simulink model "model"  (R2018b)
settings: Solver=VariableStepAuto  StartTime=0.0  StopTime=Tsim  RelTol=1e-3
values from neighbouring files (symbols this model uses):
  alfa_b_1 = -1    [init.m]
  alfa_b_3 = 0.0066    [init.m]
  b2_ref = 1.541e-5    (= 1.541e-05)    [init.m]
  b3_ref = 2.805e-2    (= 0.02805)    [init.m]
  b_0 = 1.07    [init.m]
  b_1_ref = 3.503e-3    (= 0.003503)    [init.m]
  beta_b1 = 2.157    [init.m]
  beta_c2 = 4.54    [init.m]
  c_0_ref = 75.64    [init.m]
  c_2_ref = 3.9193e-3    (= 0.0039193)    [init.m]
  d_0_ref = 75.1    [init.m]
  d_3 = 0.46    [init.m]
  E_a_b2 = -42800    [init.m]
  E_a_b3 = 42800    [init.m]
  E_a_b_1 = 35392    [init.m]
  E_a_c0 = 2224    [init.m]
  E_a_c2 = -48260    [init.m]
  E_a_d_0_1 = 4126    [init.m]
  E_a_d_0_2 = 9.752e6    (= 9752000)    [init.m]
  F = 96485    [init.m]
  gamma_b_1 = 2.472    [init.m]
  R_ug = 8.314    [init.m]
  T_ref = 298.15    [init.m]
  tau_b_3 = 5    [init.m]
  theta = 0.135    [init.m]
  U_neg_ref = 0.08    [init.m]
  V_ref = 3.7    [init.m]
undefined symbols (not defined in the file or in its folder): magnitude
settings Model: Creator=Pedro  LastModifiedBy=Pedro

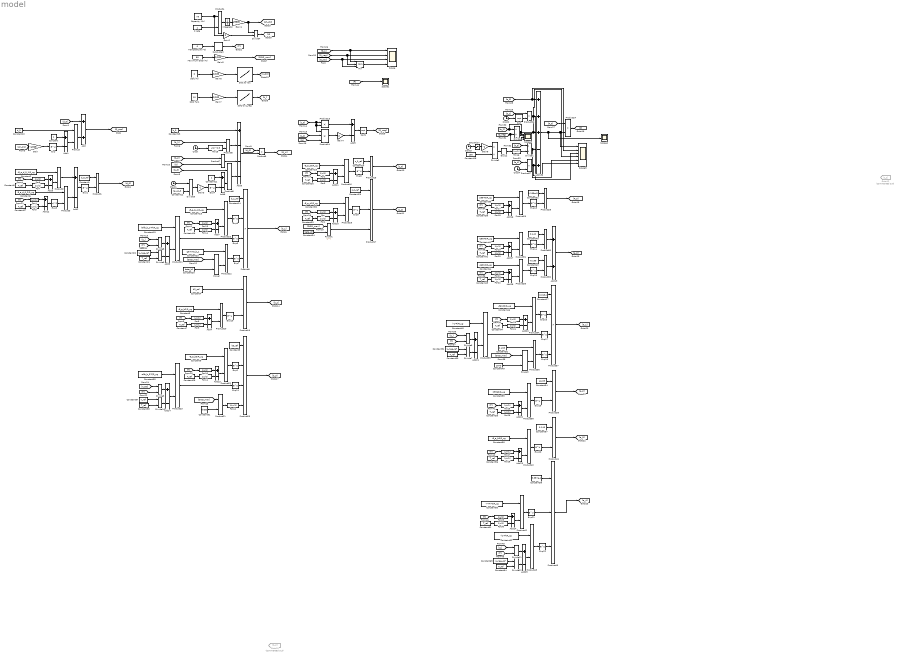
== system model ==
  Add : Sum
  Add{1..4,6..14,16..18,20..25} (22 alike) : Sum  Inputs=+-
  Add15 : Sum  Inputs=+++-+
  Add19 : Sum
  Add5 : Sum  Inputs=+---
  C rate : Constant
  Capacity (Ah) : Constant  Value=75
  Clock{,1..4} (5 alike) : Clock
  Constant : Constant
  Constant1 : Constant  Value=d_0_ref
  Constant10 : Constant  Value=d_3
  Constant11 : Constant
  Constant12 : Constant  Value=tau_b_3
  Constant13 : Constant  Value=b_0
  Constant14 : Constant  Value=b_1_ref
  Constant15 : Constant  Value=-E_a_b_1/R_ug
  Constant{3,7,16,21,26..28,33,38..39,42,45,47,50,53,56,61,64} (18 alike) : Constant  Value=T_ref
  Constant17 : Constant  Value=0.0134
  Constant18 : Constant  Value=100
  Constant19 : Constant  Value=(alfa_b_1*F)/R_ug
  Constant2 : Constant  Value=-E_a_d_0_1/R_ug
  Constant20 : Constant  Value=beta_b1
  Constant22 : Constant  Value=U_neg_ref
  Constant23 : Constant  Value=gamma_b_1
  Constant24 : Constant  Value=c_0_ref
  Constant25 : Constant  Value=-E_a_c0/R_ug  VectorParams1D=off
  Constant29 : Constant  Value=c_2_ref
  Constant30 : Constant  Value=-E_a_c2/R_ug  VectorParams1D=off
  Constant31 : Constant  Value=theta
  Constant32 : Constant  Value=1.155e-3
  Constant34 : Constant  Value=beta_c2
  Constant35 : Constant  Value=alfa_b_3*F/R_ug
  Constant36 : Constant  Value=28640/R_ug  VectorParams1D=off
  Constant37 : Constant  Value=V_ref
  Constant4 : Constant  Value=b2_ref
  Constant40 : Constant  Value=0.442
  Constant41 : Constant  Value=-28640/R_ug  VectorParams1D=off
  Constant43 : Constant  Value=-0.199
  Constant44 : Constant  Value=46010/R_ug  VectorParams1D=off
  Constant46 : Constant  Value=-36100/R_ug
  Constant48 : Constant  Value=(-1*F)/R_ug
  Constant49 : Constant  Value=1870
  Constant5 : Constant  Value=-E_a_b2/R_ug  VectorParams1D=off
  Constant51 : Constant  Value=U_neg_ref
  Constant52 : Constant  Value=2.433
  Constant54 : Constant  Value=46.05
  Constant55 : Constant  Value=29360/R_ug
  Constant57 : Constant  Value=0.145
  Constant58 : Constant  Value=-E_a_b3/R_ug
  Constant59 : Constant  Value=5.357e-4
  Constant6 : Constant  Value=E_a_d_0_2/R_ug
  Constant60 : Constant  Value=-77470/R_ug
  Constant62 : Constant  Value=(-1*F)/R_ug
  Constant65 : Constant  Value=U_neg_ref
  Constant8 : Constant  Value=b3_ref
  Constant9 : Constant  Value=-E_a_b3/R_ug
  Divide{,1..12} (13 alike) : Product  Inputs=*/
  Exp{,1..2,4..22} (22 alike) : Math  SaturateOnIntegerOverflow=on
  Exp3 : Math  Operator=magnitude^2  SaturateOnIntegerOverflow=on
  Fcn{,1..11,13..14,17..30} (28 alike) : Fcn  Expr=1/u(1)
  Fcn12 : Fcn  Expr=1+u(1)
  Fcn15 : Fcn  Expr=u(1)^0.5
  Fcn16 : Fcn  Expr=1-u(1)
  Gain : Gain  Gain=-1/228
  Gain1 : Gain  Gain=1/3600
  Gain2 : Gain  Gain=2
  Gain3 : Gain  Gain=-1
  Gain4 : Gain  Gain=2
  Gain5 : Gain  Gain=1/100
  Gain6 : Gain  Gain=1/100
  Gain7 : Gain  Gain=1/100
  Gain8 : Gain  Gain=-1
  Goto12 : Goto  Commented=on  GotoTag=c_2
  Goto15 : Goto  Commented=on  GotoTag=b_2
  Integrator : Integrator
  Maximum DOD (%) : Constant  Value=80
  Min : MinMax  Inputs=3
  Power : Math  Operator=pow  SaturateOnIntegerOverflow=on
  Power1 : Math  Operator=pow  SaturateOnIntegerOverflow=on
  Power2 : Math  Operator=pow  SaturateOnIntegerOverflow=on
  Product{,1..8,10..13,15..16,18..24,26..36,38..43} (39 alike) : Product
  Product14 : Product  Inputs=3
  Product17 : Product  Inputs=3
  Product25 : Product  Inputs=4
  Product37 : Product  Inputs=4
  Product45 : Product  Inputs=3
  Product9 : Product  Inputs=4
  SOC (%) : Constant  Value=0
  SOC (%)1 : Constant  Value=10
  SOC to U_neg : Lookup_n-D  NumberOfTableDimensions=1  BreakpointsForDimension1=[0 0.1 0.2 0.3 0.4 0.5 0.6 0.7 0.8 0.9 1.0]  Table=[1.2868 0.2420 0.1818 0.1488 0.1297 0.1230 0.1181 0.1061 0.0925 0.0876 0.0859]  InternalRulePriority=Speed  RndMeth=Simplest  InputSameDT=on
  SOC to Voc : Lookup_n-D  NumberOfTableDimensions=1  BreakpointsForDimension1=[0 0.1 0.2 0.3 0.4 0.5 0.6 0.7 0.8 0.9 1.0]  Table=[3.0000 3.4679 3.5394 3.5950 3.6453 3.6876 3.7469 3.8400 3.9521 4.0668 4.1934]  InternalRulePriority=Speed  RndMeth=Simplest  InputSameDT=on
  Saturation : Saturate  UpperLimit=inf  LowerLimit=1
  Scope : Scope  NumInputPorts=4
  Scope1 : Scope
  Scope2 : Scope
  Scope3 : Scope  NumInputPorts=3
  Scope5 : Scope  NumInputPorts=6
  Sqrt : Sqrt  SaturateOnIntegerOverflow=on
  Sqrt1 : Sqrt  SaturateOnIntegerOverflow=on
  Subsystem : Subsystem
  Temperature (°C) : Constant  Value=0
  wires:
  Constant10/1 -> Product/1
  Add1/1 -> Product/2
  Constant/1 -> Add1/1
  Exp/1 -> Add1/2
  Gain/1 -> Exp/1
  [Ah_dis] -> Gain/1
  Product/1 -> Add/2
  Add/1 -> [Q_pos]  "Positive electrode  site-limited capacity"
  Constant1/1 -> Product1/1
  Exp1/1 -> Product1/2
  Add2/1 -> Exp1/1
  Product1/1 -> [d_0]  "Increase in  capacity at BOL"
  Product2/1 -> Add2/1
  Product3/1 -> Add2/2
  Constant2/1 -> Product2/1
  Add12/1 -> Exp3/1
  Exp3/1 -> Product3/2
  [Q_pos] -> Min/3, Scope/3  "Q_pos"
  Integrator/1 -> Gain1/1
  Subsystem/1(°K) -> [T]
  Gain1/1 -> Divide4/1, [Ah_dis]
  C rate/1 -> Product4/2
  [d_0] -> Add/1
  Temperature (°C)/1 -> Subsystem/1(°C)
  Constant6/1 -> Product3/1
  Product4/1 -> Integrator/1
  Capacity (Ah)/1 -> Gain2/1, Product4/1
  Product5/1 -> [Q_Li]  "Li-limited  capacity"
  [d_0] -> Product5/1
  Add5/1 -> Product5/2
  Constant13/1 -> Add5/1
  Product6/1 -> Add5/2
  [b_1] -> Product6/1
  Fcn15/1 -> Product6/2
  Gain2/1 -> Divide4/2
  Product7/1 -> Add5/3
  [b_2] -> Product7/1
  [N] -> Product7/2
  [b_3] -> Product8/1
  Gain3/1 -> Exp4/1
  Constant11/1 -> Add6/1
  Add6/1 -> Product8/2
  Product8/1 -> Add5/4
  Exp4/1 -> Add6/2
  Divide5/1 -> Gain3/1
  Constant12/1 -> Divide5/2
  Product9/1 -> [b_1]  "SEI growth with calendar time"
  Constant14/1 -> Product9/1
  Exp5/1 -> Product9/2
  Constant15/1 -> Product10/1
  Product10/1 -> Exp5/1
  Product11/1 -> Exp6/1
  Constant21/1 -> Divide9/2
  [T] -> Divide8/2
  Constant22/1 -> Divide9/1
  Add8/1 -> Product11/2
  Constant19/1 -> Product11/1
  Divide9/1 -> Add8/2
  [U_] -> Divide8/1
  Divide8/1 -> Add8/1
  Constant23/1 -> Product12/1
  Power/1 -> Product12/2
  [DOD_max] -> Power/1
  Constant20/1 -> Power/2
  Sqrt1/1 -> [Q_neg]
  Add9/1 -> Sqrt1/1
  [c_0] -> Product14/1, Product13/2, Product13/1
  Product13/1 -> Add9/1
  Product14/1 -> Gain4/1
  [c_2] -> Product14/2
  [N] -> Product14/3
  Constant25/1 -> Product16/1
  Exp8/1 -> Product15/2
  Product15/1 -> [c_0]  "Negative electrode  site-limited capacity"
  Product16/1 -> Exp8/1
  Constant24/1 -> Product15/1
  Add10/1 -> Product18/2
  [T] -> Fcn/1
  Constant29/1 -> Product17/1
  Constant33/1 -> Fcn1/1
  Product18/1 -> Exp9/1
  Constant30/1 -> Product18/1
  Product17/1 -> [c_2]  "Capacity loss  per cycle ratio"
  [DOD_max] -> Power1/1
  Constant34/1 -> Power1/2
  Power1/1 -> Product17/3
  Divide4/1 -> [N]
  Maximum DOD (%)/1 -> Gain5/1
  Fcn/1 -> Add10/1
  Fcn1/1 -> Add10/2
  Add11/1 -> Product16/2
  Constant26/1 -> Fcn3/1
  Fcn3/1 -> Add11/2
  [T] -> Fcn2/1
  Fcn2/1 -> Add11/1
  Constant27/1 -> Fcn5/1
  Fcn5/1 -> Add12/2
  [T] -> Fcn4/1
  Fcn4/1 -> Add12/1
  Add3/1 -> Product2/2
  Constant3/1 -> Fcn7/1
  Fcn7/1 -> Add3/2
  [T] -> Fcn6/1
  Fcn6/1 -> Add3/1
  Exp9/1 -> Product17/2
  Gain5/1 -> [DOD_max]
  SOC (%)/1 -> Gain6/1
  SOC to U_neg/1 -> [U_]
  SOC to Voc/1 -> [V_OC]
  Product19/1 -> [b_2]
  Constant4/1 -> Product19/1
  Constant5/1 -> Product20/1
  Exp10/1 -> Product19/2
  Constant7/1 -> Fcn9/1
  [T] -> Fcn8/1
  Fcn9/1 -> Add4/2
  Add4/1 -> Product20/2
  Fcn8/1 -> Add4/1
  Product20/1 -> Exp10/1
  Exp2/1 -> Product25/2
  Constant9/1 -> Product22/1
  Divide3/1 -> Add14/1
  Fcn12/1 -> Product25/4
  [V_OC] -> Divide3/1
  Divide10/1 -> Add14/2
  [T] -> Divide3/2
  [DOD_max] -> Product21/1
  Exp11/1 -> Product25/3
  Constant35/1 -> Product23/1
  Product22/1 -> Exp2/1
  Product25/1 -> [b_3]  "SEI growth with calendar time"
  Constant38/1 -> Divide10/2
  Constant37/1 -> Divide10/1
  Product23/1 -> Exp11/1
  Add14/1 -> Product23/2
  Add13/1 -> Product22/2
  Fcn11/1 -> Add13/2
  Constant28/1 -> Fcn11/1
  Fcn10/1 -> Add13/1
  [T] -> Fcn10/1
  Constant8/1 -> Product25/1
  Constant31/1 -> Product21/2
  Product21/1 -> Fcn12/1
  [Q_Li] -> Min/1, Scope/1  "Q_Li"
  Exp6/1 -> Product9/3
  Add7/1 -> Product10/2
  Fcn13/1 -> Add7/1
  Constant16/1 -> Fcn14/1
  Fcn14/1 -> Add7/2
  [T] -> Fcn13/1
  Clock/1 -> Fcn15/1
  Clock1/1 -> Divide5/1
  Exp7/1 -> Product9/4
  SOC (%)1/1 -> Gain7/1
  Gain7/1 -> SOC to U_neg/1
  Gain6/1 -> SOC to Voc/1
  [Q_neg] -> Min/2, Scope/2  "Q_neg"
  Min/1 -> Scope/4
  Product24/1 -> [R]
  [R_0] -> Product24/1
  Add15/1 -> Scope2/1, Scope5/1, Product24/2  "Result"
  [a_0] -> Scope5/2, Add15/1  "+"
  Clock2/1 -> Sqrt/1
  Product26/1 -> Scope5/3, Add15/2  "+"
  [a_1] -> Product26/1
  Sqrt/1 -> Product26/2
  Divide/1 -> Scope3/3, Scope5/4, Add15/3  "+"
  [Q_neg] -> Scope3/2, Divide/2  "Q_neg"
  [a_3] -> Divide1/1
  Divide1/1 -> Scope5/5, Add15/4  "-"
  Fcn16/1 -> Divide1/2
  Exp12/1 -> Fcn16/1
  Divide2/1 -> Exp12/1
  Gain8/1 -> Divide2/1
  Constant18/1 -> Divide2/2
  Product27/1 -> Scope5/6, Add15/5  "+"
  Clock4/1 -> Product27/2
  [a_4] -> Product27/1
  Add16/1 -> Product29/2
  Constant32/1 -> Product28/1
  Product28/1 -> [R_0]  "Instantaneous  temperature response"
  Fcn18/1 -> Add16/2
  Constant36/1 -> Product29/1
  Product29/1 -> Exp13/1
  Fcn17/1 -> Add16/1
  Exp13/1 -> Product28/2
  [T] -> Fcn17/1
  Constant39/1 -> Fcn18/1
  Add17/1 -> Product31/2
  Fcn19/1 -> Add17/1
  Fcn20/1 -> Add17/2
  Constant41/1 -> Product31/1
  Product31/1 -> Exp14/1
  Product30/1 -> Add19/1
  Constant40/1 -> Product30/1
  Exp14/1 -> Product30/2
  [T] -> Fcn19/1
  Constant42/1 -> Fcn20/1
  Constant43/1 -> Product32/1
  Product32/1 -> Add19/2
  Exp15/1 -> Product32/2
  Constant45/1 -> Fcn22/1
  Fcn21/1 -> Add18/1
  Fcn22/1 -> Add18/2
  Product33/1 -> Exp15/1
  Add18/1 -> Product33/2
  Constant44/1 -> Product33/1
  [T] -> Fcn21/1
  Add19/1 -> [a_0]  "Base  resistance"
  Product12/1 -> Exp7/1
  [T] -> Fcn23/1
  Fcn24/1 -> Add20/2
  Fcn23/1 -> Add20/1
  Exp17/1 -> Product37/3
  Power2/1 -> Product36/2
  Constant51/1 -> Divide7/1
  Constant47/1 -> Fcn24/1
  Exp16/1 -> Product37/2
  Divide6/1 -> Add21/1
  Constant49/1 -> Power2/2
  Constant50/1 -> Divide7/2
  Add21/1 -> Product35/2
  [DOD_max] -> Power2/1
  Constant17/1 -> Product37/1
  Divide7/1 -> Add21/2
  Product35/1 -> Exp17/1
  Exp18/1 -> Product37/4
  Constant52/1 -> Product36/1
  Product37/1 -> [a_1]  "SEI growth with calendar time"
  [T] -> Divide6/2
  Add20/1 -> Product34/2
  [U_] -> Divide6/1
  Constant48/1 -> Product35/1
  Constant46/1 -> Product34/1
  Product36/1 -> Exp18/1
  Product34/1 -> Exp16/1
  Constant53/1 -> Fcn26/1
  Exp19/1 -> Product39/2
  Constant54/1 -> Product39/1
  Add22/1 -> Product38/2
  [T] -> Fcn25/1
  Fcn26/1 -> Add22/2
  Product39/1 -> [a_2]  "Loss with cycling"
  Fcn25/1 -> Add22/1
  Constant55/1 -> Product38/1
  Product38/1 -> Exp19/1
  Fcn28/1 -> Add23/2
  Constant58/1 -> Product40/1
  Constant57/1 -> Product41/1
  Product41/1 -> [a_3]  "Break-in mechanism at BOL"
  Exp20/1 -> Product41/2
  Add23/1 -> Product40/2
  Fcn27/1 -> Add23/1
  Product40/1 -> Exp20/1
  [T] -> Fcn27/1
  Constant56/1 -> Fcn28/1
  Fcn30/1 -> Add24/2
  [T] -> Fcn29/1
  Fcn29/1 -> Add24/1
  Divide11/1 -> Add25/1
  Constant61/1 -> Fcn30/1
  Exp22/1 -> Product45/3
  Constant64/1 -> Divide12/2
  Product42/1 -> Exp21/1
  Constant60/1 -> Product42/1
  Constant62/1 -> Product43/1
  [U_] -> Divide11/1
  Add24/1 -> Product42/2
  Product43/1 -> Exp22/1
  Divide12/1 -> Add25/2
  Constant59/1 -> Product45/1
  Constant65/1 -> Divide12/1
  [T] -> Divide11/2
  Exp21/1 -> Product45/2
  Add25/1 -> Product43/2
  Product45/1 -> [a_4]  "SEI growth with calendar time"
  [R] -> Scope1/1  "R"
  Clock3/1 -> Saturation/1
  Saturation/1 -> Gain8/1
  [a_2] -> Scope3/1, Divide/1
  Gain4/1 -> Add9/2

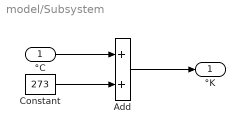
== system model/Subsystem ==
  °C : Inport
  Add : Sum
  Constant : Constant  Value=273
  °K : Outport
  wires:
  Constant/1 -> Add/2
  °C/1 -> Add/1
  Add/1 -> °K/1
